simulink model "test_fft"  (R2012b)
settings: Solver=ode45  StartTime=0.0  StopTime=10.0  RelTol=1e-3
libraries: xbsIndex_r4 x6538, casper_library_misc x220, casper_library_delays x31, xbsReplacements_r4 x4, casper_library_ffts_twiddle x2, simulink x1
(part 59 of 104)

== system test_fft/fft0/fft_direct/butterfly3_3/twiddle_general_4mult/coeff_gen ==
  rst : Inport
  Counter : xbsIndex_r4/Counter  cnt_type=Free Running  cnt_to=Inf  operation=Up  start_count=0  cnt_by_val=1  arith_type=Unsigned  n_bits=12  bin_pt=0  load_pin=off  rst=on  en=off  explicit_period=on  period=1  dbl_ovrd=off  use_behavioral_HDL=off  implementation=Fabric  block_type=counter
  ROM : xbsIndex_r4/ROM  depth=4096  initVector="[-0.7071075439453125                     -0.707244873046875                    -0.7073822021484375                         -0.70751953125                       -0.7076416015625                    -0.7077789306640625                     -0.707916259765625                    -0.7080535888671875                      -0.70819091796875                    -0.7083282470703125                     -0.708465576171875                    -0.7086029052734375                    -0.7087249755859375                       -0.7088623046875                    -0.7089996337890625                     -0.709136962890625                    -0.7092742919921875                      -0.70941162109375                    -0.7095489501953125                    -0.7096710205078125                     -0.709808349609375                    -0.7099456787109375                       -0.7100830078125                    -0.7102203369140625                     -0.710357666015625                    -0.7104949951171875                    -0.7106170654296875                      -0.71075439453125                    -0.7108917236328125                     -0.711029052734375                    -0.7111663818359375                       -0.7113037109375                         -0.71142578125                    -0.7115631103515625                     -0.711700439453125                    -0.7118377685546875                      -0.71197509765625                    -0.7121124267578125                    -0.7122344970703125                     -0.712371826171875                    -0.7125091552734375                        -0.712646484375                    -0.7127838134765625                    -0.7129058837890625                     -0.713043212890625                    -0.7131805419921875                      -0.71331787109375                    -0.7134552001953125                    -0.7135772705078125                     -0.713714599609375                    -0.7138519287109375                       -0.7139892578125                    -0.7141265869140625                    -0.7142486572265625                     -0.714385986328125                    -0.7145233154296875                      -0.71466064453125                    -0.7147979736328125                    -0.7149200439453125                     -0.715057373046875                    -0.7151947021484375                         -0.71533203125                    -0.7154693603515625                    -0.7155914306640625                     -0.715728759765625                    -0.7158660888671875                      -0.71600341796875                      -0.71612548828125                    -0.7162628173828125                     -0.716400146484375                    -0.7165374755859375                       -0.7166748046875                           -0.716796875                    -0.7169342041015625                     -0.717071533203125                    -0.7172088623046875                    -0.7173309326171875                      -0.71746826171875                    -0.7176055908203125                     -0.717742919921875                     -0.717864990234375                    -0.7180023193359375                       -0.7181396484375                    -0.7182769775390625                    -0.7183990478515625                     -0.718536376953125                    -0.7186737060546875                      -0.71881103515625                      -0.71893310546875                    -0.7190704345703125                     -0.719207763671875                     -0.719329833984375                    -0.7194671630859375                       -0.7196044921875                    -0.7197418212890625                    -0.7198638916015625                     -0.720001220703125                    -0.7201385498046875                      -0.72027587890625                      -0.72039794921875                    -0.7205352783203125                     -0.720672607421875                     -0.720794677734375 ...(+155726 chars)]"  distributed_mem=Block RAM  rst=off  init_reg=0  en=off  latency=4  gui_display_data_type=Fixed-point  arith_type="Signed  (2's comp)"  n_bits=18  bin_pt=16  preci_type=Single  exp_width=8  frac_width=24  dbl_ovrd=off  optimize=Area  use_rpm=on  block_type=sprom
  ROM1 : xbsIndex_r4/ROM  depth=4096  initVector="[-0.7071075439453125                      -0.70697021484375                    -0.7068328857421875                     -0.706695556640625                    -0.7065582275390625                       -0.7064208984375                        -0.706298828125                    -0.7061614990234375                     -0.706024169921875                    -0.7058868408203125                      -0.70574951171875                    -0.7056121826171875                     -0.705474853515625                    -0.7053375244140625                       -0.7052001953125                    -0.7050628662109375                    -0.7049407958984375                     -0.704803466796875                    -0.7046661376953125                      -0.70452880859375                    -0.7043914794921875                     -0.704254150390625                    -0.7041168212890625                       -0.7039794921875                    -0.7038421630859375                     -0.703704833984375                    -0.7035675048828125                      -0.70343017578125                    -0.7032928466796875                    -0.7031707763671875                     -0.703033447265625                    -0.7028961181640625                       -0.7027587890625                    -0.7026214599609375                     -0.702484130859375                    -0.7023468017578125                      -0.70220947265625                    -0.7020721435546875                     -0.701934814453125                    -0.7017974853515625                         -0.70166015625                    -0.7015228271484375                     -0.701385498046875                    -0.7012481689453125                      -0.70111083984375                    -0.7009735107421875                     -0.700836181640625                    -0.7006988525390625                       -0.7005615234375                        -0.700439453125                    -0.7003021240234375                     -0.700164794921875                    -0.7000274658203125                      -0.69989013671875                    -0.6997528076171875                     -0.699615478515625                    -0.6994781494140625                       -0.6993408203125                    -0.6992034912109375                     -0.699066162109375                    -0.6989288330078125                      -0.69879150390625                    -0.6986541748046875                     -0.698516845703125                    -0.6983795166015625                          -0.6982421875                    -0.6981048583984375                     -0.697967529296875                    -0.6978302001953125                      -0.69769287109375                    -0.6975555419921875                     -0.697418212890625                    -0.6972808837890625                       -0.6971435546875                    -0.6970062255859375                     -0.696868896484375                    -0.6967315673828125                      -0.69659423828125                    -0.6964569091796875                     -0.696319580078125                    -0.6961822509765625                        -0.696044921875                    -0.6959075927734375                     -0.695770263671875                    -0.6956329345703125                      -0.69549560546875                    -0.6953582763671875                    -0.6952056884765625                        -0.695068359375                    -0.6949310302734375                     -0.694793701171875                    -0.6946563720703125                      -0.69451904296875                    -0.6943817138671875                     -0.694244384765625                    -0.6941070556640625                       -0.6939697265625                    -0.6938323974609375                     -0.693695068359375                    -0.6935577392578125                      -0.69342041015625                    -0.6932830810546875                     -0.693145751953125 ...(+155726 chars)]"  distributed_mem=Block RAM  rst=off  init_reg=0  en=off  latency=4  gui_display_data_type=Fixed-point  arith_type="Signed  (2's comp)"  n_bits=18  bin_pt=16  preci_type=Single  exp_width=8  frac_width=24  dbl_ovrd=off  optimize=Area  use_rpm=on  block_type=sprom
  Slice : xbsIndex_r4/Slice  nbits=12  boolean_output=off  mode=Upper Bit Location + Width  bit1=0  base1=MSB of Input  bit0=0  base0=LSB of Input  dbl_ovrd=off  block_type=slice
  ri_to_c : casper_library_misc/ri_to_c
  w : Outport
  wires:
  ri_to_c/1 -> w/1
  rst/1 -> Counter/1
  Counter/1 -> Slice/1
  Slice/1 -> ROM/1, ROM1/1
  ROM/1 -> ri_to_c/1
  ROM1/1 -> ri_to_c/2
